simulink model "schema_without_atomic"  (R2013b)
settings: Solver=FixedStepDiscrete  StartTime=0.0  StopTime=0.0149  FixedStep=Te  RelTol=1e-3
values from neighbouring files (symbols this model uses):
  a0_pi = -1    [script.m]
  a0_s = 0.5488    [script.m]
  a1_pi = 1    [script.m]
  a1_s = -1.4816    [script.m]
  a2_s = 1    [script.m]
  b0_pi = -0.1750    (= -0.175)    [script.m]
  b0_s = 0.0302    [script.m]
  b1_pi = 0.25    [script.m]
  b1_s = 0.0369    [script.m]
  Te = 1e-4    (= 0.0001)    [script.m]
settings Model: Creator=gemsdev  LastModifiedBy=gemsdev
settings DataIOCC: ExternalInput=[t, x]  LoadExternalInput=on

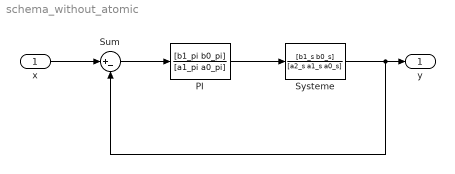
== system schema_without_atomic ==
  x : Inport
  PI : DiscreteTransferFcn  Numerator=[b1_pi b0_pi]  Denominator=[a1_pi a0_pi]  SampleTime=Te
  Sum : Sum  Inputs=|+-
  Systeme : DiscreteTransferFcn  Numerator=[b1_s b0_s]  Denominator=[a2_s a1_s a0_s]  SampleTime=Te
  y : Outport
  wires:
  PI/1 -> Systeme/1
  x/1 -> Sum/1
  Sum/1 -> PI/1
  Systeme/1 -> y/1, Sum/2
